simulink model "caidalibre"  (R2014a)
settings: Solver=ode45  StartTime=0.0  StopTime=20  RelTol=1e-3
undefined symbols (not defined in the file): g, h_inicial, k, m
libraries: simulink x2
settings Model: Creator=Manuel  LastModifiedBy=Manuel

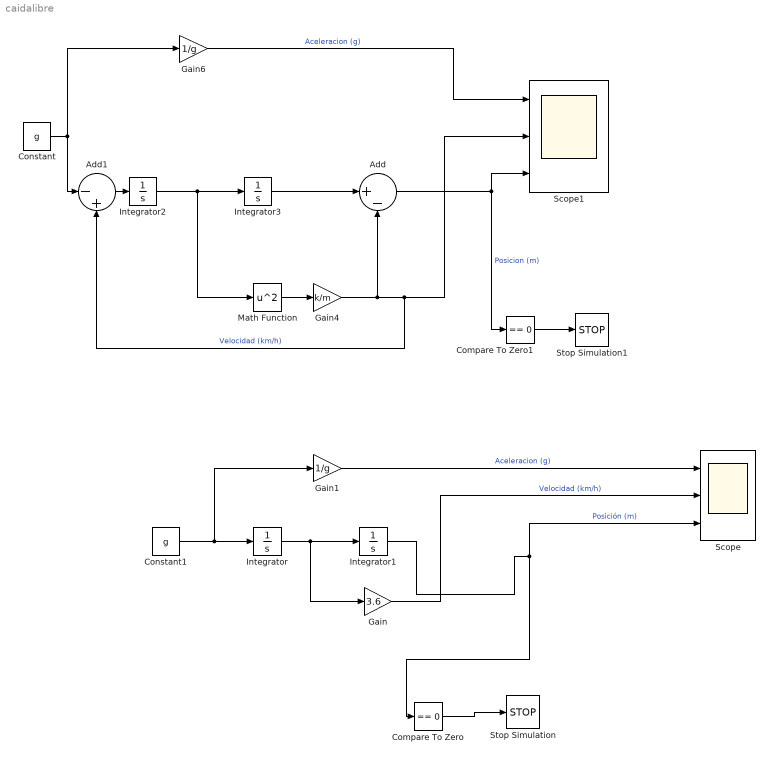
== system caidalibre ==
  Add : Sum  Inputs=|+-
  Add1 : Sum  Inputs=|-+
  Compare To Zero : simulink/Logic and Bit Operations/Compare To Zero  relop===  OutDataTypeStr=boolean
  Compare To Zero1 : simulink/Logic and Bit Operations/Compare To Zero  relop===  OutDataTypeStr=boolean
  Constant : Constant  Value=g
  Constant1 : Constant  Value=g
  Gain : Gain  Gain=3.6
  Gain1 : Gain  Gain=1/g
  Gain4 : Gain  Gain=k/m
  Gain6 : Gain  Gain=1/g
  Integrator : Integrator
  Integrator1 : Integrator  InitialCondition=h_inicial
  Integrator2 : Integrator
  Integrator3 : Integrator  InitialCondition=h_inicial
  Math Function : Math  Operator=square  SaturateOnIntegerOverflow=on
  Scope : Scope  NumInputPorts=3
      settings: ShowLegends=on  YMin=-5~-5~-5  YMax=5~5~5
  Scope1 : Scope  NumInputPorts=3
      settings: ShowLegends=on  TimeRange=6  YMin=0~0~-6e+183  YMax=2~6e+183~9.999999999999998e+182
  Stop Simulation : Stop
  Stop Simulation1 : Stop
  wires:
  Constant1/1 -> Gain1/1, Integrator/1
  Integrator/1 -> Gain/1, Integrator1/1
  Integrator1/1 -> Compare To Zero/1, Scope/3  "Posición (m)"
  Gain/1 -> Scope/2  "Velocidad (km/h)"
  Gain1/1 -> Scope/1  "Aceleracion (g)"
  Compare To Zero/1 -> Stop Simulation/1
  Constant/1 -> Add1/1, Gain6/1
  Integrator2/1 -> Math Function/1, Integrator3/1
  Add/1 -> Scope1/3, Compare To Zero1/1  "Posicion (m)"
  Math Function/1 -> Gain4/1
  Compare To Zero1/1 -> Stop Simulation1/1
  Gain4/1 -> Add1/2, Scope1/2, Add/2  "Velocidad (km/h)"
  Gain6/1 -> Scope1/1  "Aceleracion (g)"
  Integrator3/1 -> Add/1
  Add1/1 -> Integrator2/1
